simulink model "opt_lab11_Kalman_sim"  (R2018a)
settings: Solver=VariableStepAuto  StartTime=0.0  StopTime=t(end)  RelTol=1e-3
values from neighbouring files (symbols this model uses):
  Ad = [0.16   -0.4002   -0.478 ... (first row only)    [gyak11.m]
  Bd = [0.0390 0.1 ... (first row only)    [gyak11.m]
  Cd = [1 2 -1]    [gyak11.m]
  K = Ptemp*Cd'*inv(Cd*Ptemp*Cd'+R)    [gyak11.m]
  Ts = 0.1    [gyak11.m]
  x0 = [2 4 1]'    [gyak11.m]
settings Model: Creator=Sandor Matyas  LastModifiedBy=alfac

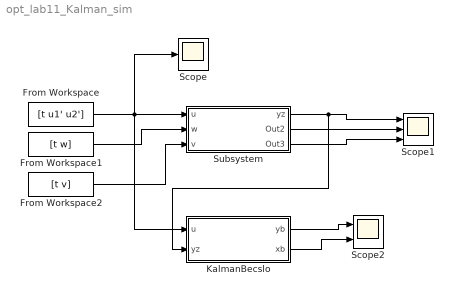
== system opt_lab11_Kalman_sim ==
  From Workspace : FromWorkspace  VariableName=[t u1' u2']  SampleTime=Ts
  From Workspace1 : FromWorkspace  VariableName=[t w]  SampleTime=Ts
  From Workspace2 : FromWorkspace  VariableName=[t v]  SampleTime=Ts
  KalmanBecslo : Subsystem
  Scope : Scope
  Scope1 : Scope  NumInputPorts=3
  Scope2 : Scope  NumInputPorts=2
  Subsystem : Subsystem
  wires:
  From Workspace/1 -> KalmanBecslo/1(u), Subsystem/1("u "), Scope/1
  From Workspace1/1 -> Subsystem/2(w)
  From Workspace2/1 -> Subsystem/3(v)
  Subsystem/1(yz) -> KalmanBecslo/2(yz), Scope1/1
  Subsystem/2(Out2) -> Scope1/2
  Subsystem/3(Out3) -> Scope1/3
  KalmanBecslo/1(yb) -> Scope2/1
  KalmanBecslo/2(xb) -> Scope2/2

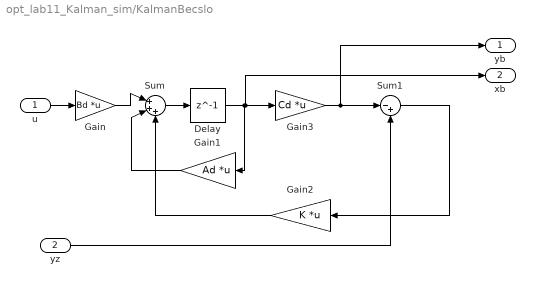
== system opt_lab11_Kalman_sim/KalmanBecslo ==
  u : Inport
  yz : Inport  Port=2
  Delay : Delay  DelayLength=1  InitialCondition=0
  Gain : Gain  Gain=Bd  Multiplication=Matrix(K*u)
  Gain1 : Gain  Gain=Ad  Multiplication=Matrix(K*u)
  Gain2 : Gain  Gain=K  Multiplication=Matrix(K*u)
  Gain3 : Gain  Gain=Cd  Multiplication=Matrix(K*u)
  Sum : Sum  Inputs=|+++
  Sum1 : Sum  Inputs=|-+
  yb : Outport
  xb : Outport  Port=2
  wires:
  Gain/1 -> Sum/1
  Gain1/1 -> Sum/2
  Sum/1 -> Delay/1
  Delay/1 -> Gain1/1, xb/1, Gain3/1
  Gain3/1 -> yb/1, Sum1/1
  yz/1 -> Sum1/2
  Sum1/1 -> Gain2/1
  Gain2/1 -> Sum/3
  u/1 -> Gain/1

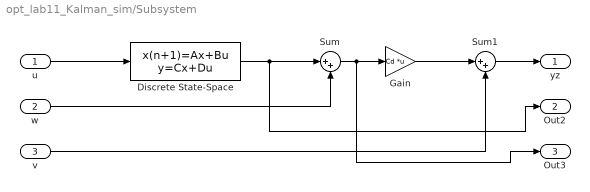
== system opt_lab11_Kalman_sim/Subsystem ==
  "u " : Inport
  w : Inport  Port=2
  v : Inport  Port=3
  Discrete State-Space : DiscreteStateSpace  A=Ad  B=Bd  C=eye(3)  D=zeros(3,2)  InitialCondition=x0  SampleTime=Ts
  Gain : Gain  Gain=Cd  Multiplication=Matrix(K*u)
  Sum : Sum  Inputs=|++
  Sum1 : Sum  Inputs=|++
  yz : Outport
  Out2 : Outport  Port=2
  Out3 : Outport  Port=3
  wires:
  Discrete State-Space/1 -> Out2/1, Sum/1
  Sum/1 -> Out3/1, Gain/1
  "u "/1 -> Discrete State-Space/1
  w/1 -> Sum/2
  v/1 -> Sum1/2
  Gain/1 -> Sum1/1
  Sum1/1 -> yz/1
